simulink model "set_nav420_to_quiet_standalone_model"  (Simulink 7.4)
settings: Solver=ode3  StartTime=0.0  StopTime=inf  RelTol=1e-3
undefined symbols (not defined in the file or in its folder): serial
libraries: instrumentlib x1
settings Model: Creator=djulzz  LastModifiedBy=autopilot

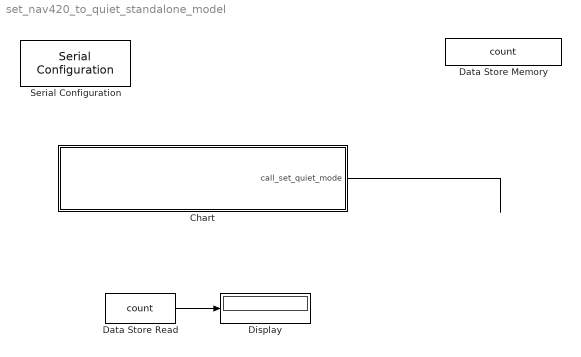
== system set_nav420_to_quiet_standalone_model ==
  Chart : Stateflow chart
  Data Store Memory : DataStoreMemory  DataStoreName=count  DataType=uint8  OutDataType=fixdt(1, 16)  OutScaling=2^0  OutDataTypeStr=uint8
  Data Store Read : DataStoreRead  DataStoreName=count  SampleTime=-1
  Display : Display
      settings: Format=hex (Stored Integer)
  Serial Configuration : instrumentlib/Serial Configuration  Priority=-200000  DialogController=instrumentcreatedialog  DialogControllerArgs=DataTag0  ComPortMenu=COM1  ComPort=COM1  ObjConstructor=serial('COM1');  BaudRate=38400  DataBits=8  Parity=none  StopBits=1  FlowControl=none  Timeout=10  ByteOrder=LittleEndian
  wires:
  Data Store Read/1 -> Display/1
  Chart/1(call_set_quiet_mode) -> ?

== stateflow chart Chart ==
  state Step1
    count=0;
    call_set_quiet_mode=1;
  state End
  (default) -> Step1
  Step1 -> End
  data: count data_store_memory double; call_set_quiet_mode output uint8
